simulink model "sim_4"  (R2021a)
settings: Solver=VariableStepAuto  StartTime=0.0  StopTime=25  RelTol=1e-3
libraries: cstblocks x12
settings Model: Creator=me-clab2  LastModifiedBy=HASEE
settings SolverCC: AlgebraicLoopSolver=TrustRegion
settings DebuggingCC: SFMachineParentedDataDiag=warning

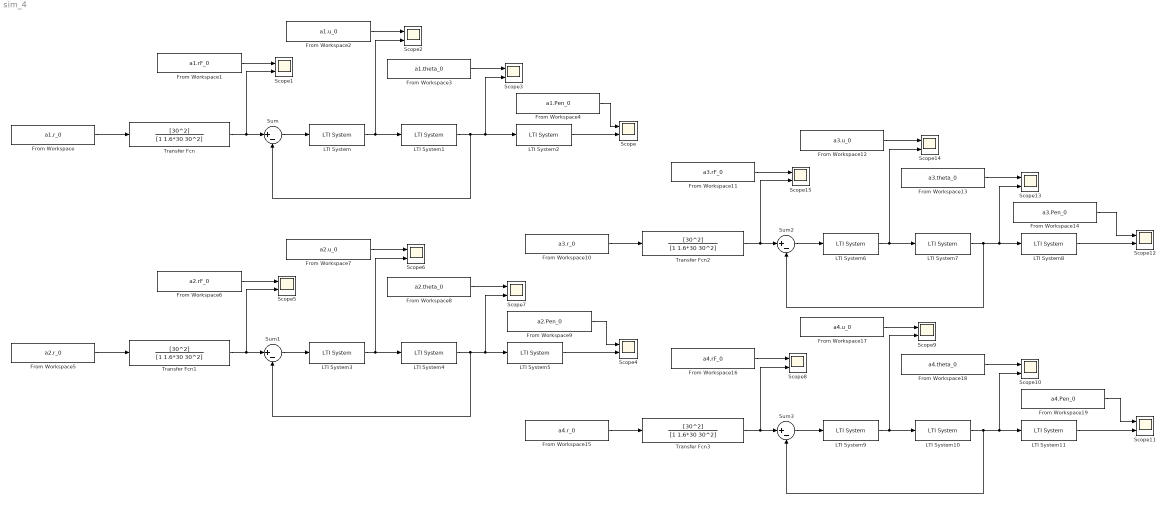
== system sim_4 ==
  From Workspace : FromWorkspace  VariableName=a1.r_0
  From Workspace1 : FromWorkspace  VariableName=a1.rF_0
  From Workspace10 : FromWorkspace  VariableName=a3.r_0
  From Workspace11 : FromWorkspace  VariableName=a3.rF_0
  From Workspace12 : FromWorkspace  VariableName=a3.u_0
  From Workspace13 : FromWorkspace  VariableName=a3.theta_0
  From Workspace14 : FromWorkspace  VariableName=a3.Pen_0
  From Workspace15 : FromWorkspace  VariableName=a4.r_0
  From Workspace16 : FromWorkspace  VariableName=a4.rF_0
  From Workspace17 : FromWorkspace  VariableName=a4.u_0
  From Workspace18 : FromWorkspace  VariableName=a4.theta_0
  From Workspace19 : FromWorkspace  VariableName=a4.Pen_0
  From Workspace2 : FromWorkspace  VariableName=a1.u_0
  From Workspace3 : FromWorkspace  VariableName=a1.theta_0
  From Workspace4 : FromWorkspace  VariableName=a1.Pen_0
  From Workspace5 : FromWorkspace  VariableName=a2.r_0
  From Workspace6 : FromWorkspace  VariableName=a2.rF_0
  From Workspace7 : FromWorkspace  VariableName=a2.u_0
  From Workspace8 : FromWorkspace  VariableName=a2.theta_0
  From Workspace9 : FromWorkspace  VariableName=a2.Pen_0
  LTI System : cstblocks/LTI System  sys=0.02  IC=[]
  LTI System{1,4,7,10} (4 alike) : cstblocks/LTI System  sys=Py  IC=[]
  LTI System{2,5,8,11} (4 alike) : cstblocks/LTI System  sys=Pt  IC=[]
  LTI System3 : cstblocks/LTI System  sys=C2  IC=[]
  LTI System6 : cstblocks/LTI System  sys=C2  IC=[]
  LTI System9 : cstblocks/LTI System  sys=C2  IC=[]
  Scope{,1..15} (16 alike) : Scope  NumInputPorts=2
  Sum{,1..3} (4 alike) : Sum  Inputs=|+-
  Transfer Fcn{,1..3} (4 alike) : TransferFcn  Numerator=[30^2]  Denominator=[1 1.6*30 30^2]
  wires:
  Transfer Fcn/1 -> Scope1/2, Sum/1
  Sum/1 -> LTI System/1
  From Workspace/1 -> Transfer Fcn/1
  From Workspace1/1 -> Scope1/1
  LTI System/1 -> Scope2/2, LTI System1/1
  From Workspace2/1 -> Scope2/1
  LTI System1/1 -> Scope3/2, LTI System2/1, Sum/2
  From Workspace3/1 -> Scope3/1
  From Workspace7/1 -> Scope6/1
  From Workspace6/1 -> Scope5/1
  From Workspace9/1 -> Scope4/1
  LTI System5/1 -> Scope4/2
  LTI System3/1 -> Scope6/2, LTI System4/1
  Transfer Fcn1/1 -> Scope5/2, Sum1/1
  Sum1/1 -> LTI System3/1
  From Workspace8/1 -> Scope7/1
  LTI System4/1 -> Scope7/2, LTI System5/1, Sum1/2
  From Workspace5/1 -> Transfer Fcn1/1
  From Workspace12/1 -> Scope14/1
  From Workspace11/1 -> Scope15/1
  From Workspace14/1 -> Scope12/1
  LTI System8/1 -> Scope12/2
  LTI System6/1 -> Scope14/2, LTI System7/1
  Transfer Fcn2/1 -> Scope15/2, Sum2/1
  Sum2/1 -> LTI System6/1
  From Workspace13/1 -> Scope13/1
  LTI System7/1 -> Scope13/2, LTI System8/1, Sum2/2
  From Workspace10/1 -> Transfer Fcn2/1
  From Workspace17/1 -> Scope9/1
  From Workspace16/1 -> Scope8/1
  From Workspace19/1 -> Scope11/1
  LTI System11/1 -> Scope11/2
  LTI System9/1 -> Scope9/2, LTI System10/1
  Transfer Fcn3/1 -> Scope8/2, Sum3/1
  Sum3/1 -> LTI System9/1
  From Workspace18/1 -> Scope10/1
  LTI System10/1 -> Scope10/2, LTI System11/1, Sum3/2
  From Workspace15/1 -> Transfer Fcn3/1
  LTI System2/1 -> Scope/2
  From Workspace4/1 -> Scope/1
